simulink model "PBR_process_prod"  (R2021b)
settings: Solver=VariableStepAuto  StartTime=0.0  StopTime=300  RelTol=1e-3
values from neighbouring files (symbols this model uses):
  b = 0.0008    [PBR_estim_5_param.m]    (also in PBR_optim_orizont.m)
  D = 0    [PBR_estim_5_param.m]    (also in PBR_optim_orizont.m = linspace(0,0.1,100))
  Ea = 200    [PBR_estim_5_param.m]    (also in PBR_optim_orizont.m)
  Es = 870    [PBR_estim_5_param.m]    (also in PBR_optim_orizont.m)
  I0 = 500    [PBR_estim_5_param.m]    (also in PBR_optim_orizont.m)
  Kn = params(3)    [PBR_estim_5_param.m]    (also in PBR_optim_orizont.m = 0.13236)
  Ks = params(2)    [PBR_estim_5_param.m]    (also in PBR_optim_orizont.m = 101.2637)
  L = 0.054    [PBR_estim_5_param.m]    (also in PBR_optim_orizont.m)
  mud = params(5)    [PBR_estim_5_param.m]    (also in PBR_optim_orizont.m = 0.010177)
  mumax = params(1)    [PBR_estim_5_param.m]    (also in PBR_optim_orizont.m = 0.21692)
  N0 = 2    [PBR_estim_5_param.m]    (also in PBR_optim_orizont.m = 1.5)
  Nin = 1    [PBR_estim_5_param.m]    (also in PBR_optim_orizont.m = 2)
  X0 = 0.1    [PBR_estim_5_param.m]    (also in PBR_optim_orizont.m)
  Ynx = params(4)    [PBR_estim_5_param.m]    (also in PBR_optim_orizont.m = 0.043508)
settings Model: Creator=georg
settings SolverCC: AlgebraicLoopSolver=TrustRegion
settings DataIOCC: ReturnWorkspaceOutputs=off
settings DebuggingCC: ArithmeticOperatorsInVariantConditions=warning
settings SFSimCC: CustomCodeUndefinedFunction=UseInterfaceOnly
settings RTWCC: DLArmComputeVersion=20.02.1

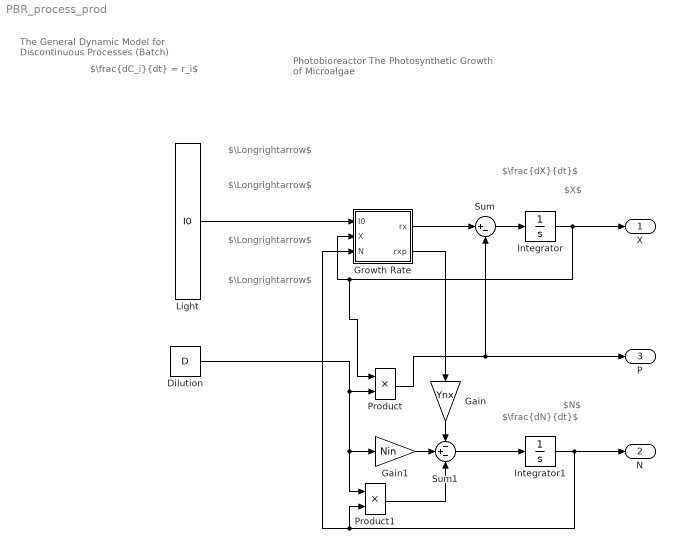
== system PBR_process_prod ==
  note: Photobioreactor
      | The Photosynthetic Growth of Microalgae
  note: $X$
  note: $\frac{dX}{dt}$
  note: $\Longrightarrow$
  note: $\Longrightarrow$
  note: $\frac{dC_i}{dt} = r_i$
  note: $\Longrightarrow$
  note: The General Dynamic Model for
      | Discontinuous Processes (Batch)
  note: $\Longrightarrow$
  note: $\frac{dN}{dt}$
  note: $N$
  Dilution : Constant  Value=D
  Gain : Gain  Gain=Ynx
  Gain1 : Gain  Gain=Nin
  Growth Rate : Subsystem
  Integrator : Integrator  InitialCondition=X0
  Integrator1 : Integrator  InitialCondition=N0
  Light : Constant  Value=I0
  Product : Product
  Product1 : Product
  Sum : Sum  Inputs=|+-
  Sum1 : Sum  Inputs=-+-
  X : Outport
  N : Outport  Port=2
  P : Outport  Port=3
  wires:
  Sum/1 -> Integrator/1
  Integrator/1 -> X/1, Growth Rate/2(X), Product/1
  Growth Rate/1(rx) -> Sum/1
  Gain1/1 -> Sum1/2
  Product1/1 -> Sum1/3
  Integrator1/1 -> N/1, Growth Rate/3(N), Product1/2
  Sum1/1 -> Integrator1/1
  Gain/1 -> Sum1/1
  Growth Rate/2(rxp) -> Gain/1
  Light/1 -> Growth Rate/1(I0)
  Dilution/1 -> Gain1/1, Product1/1, Product/2
  Product/1 -> P/1, Sum/2

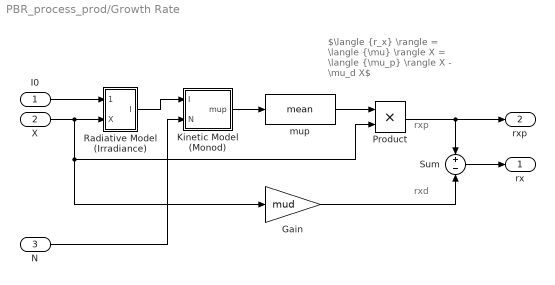
== system PBR_process_prod/Growth Rate ==
  note: $\langle {r_x} \rangle = \langle {\mu} \rangle X = \langle {\mu_p} \rangle X - \mu_d X$
  note: rxd
  note: rxp
  I0 : Inport
  X : Inport  Port=2
  N : Inport  Port=3
  Gain : Gain  Gain=mud
  Kinetic Model (Monod) : Subsystem
  Product : Product
  Radiative Model (Irradiance) : Subsystem
  Sum : Sum  Inputs=+-
  mup : MATLABFcn  MATLABFcn=mean
  rx : Outport  VectorParamsAs1DForOutWhenUnconnected=off
  rxp : Outport  Port=2  VectorParamsAs1DForOutWhenUnconnected=off
  wires:
  X/1 -> Product/2, Gain/1, Radiative Model (Irradiance)/2(X)
  Gain/1 -> Sum/2
  Sum/1 -> rx/1
  I0/1 -> Radiative Model (Irradiance)/1(I0)
  Kinetic Model (Monod)/1(mup) -> mup/1
  Radiative Model (Irradiance)/1(I) -> Kinetic Model (Monod)/1(I)
  mup/1 -> Product/1
  Product/1 -> Sum/1, rxp/1
  N/1 -> Kinetic Model (Monod)/2(N)

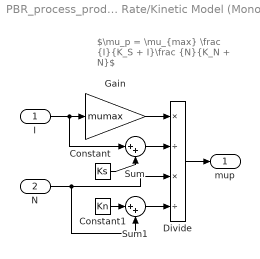
== system PBR_process_prod/Growth Rate/Kinetic Model (Monod) ==
  note: $\mu_p = \mu_{max} \frac {I}{K_S + I}\frac {N}{K_N + N}$
  I : Inport
  N : Inport  Port=2
  Constant : Constant  Value=Ks
  Constant1 : Constant  Value=Kn
  Divide : Product  Inputs=*/*/
  Gain : Gain  Gain=mumax
  Sum : Sum  Inputs=|++
  Sum1 : Sum  Inputs=|++
  mup : Outport  VectorParamsAs1DForOutWhenUnconnected=off
  wires:
  Constant/1 -> Sum/2
  Sum/1 -> Divide/2
  I/1 -> Sum/1, Gain/1
  Gain/1 -> Divide/1
  Divide/1 -> mup/1
  N/1 -> Sum1/2, Divide/3
  Sum1/1 -> Divide/4
  Constant1/1 -> Sum1/1

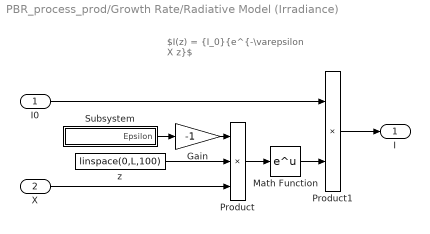
== system PBR_process_prod/Growth Rate/Radiative Model (Irradiance) ==
  note: $I(z) = {I_0}{e^{-\varepsilon X z}$
  I0 : Inport
  X : Inport  Port=2
  Gain : Gain  Gain=-1
  Math Function : Math  SignedPower=on  SaturateOnIntegerOverflow=on
  Product : Product  Inputs=3
  Product1 : Product
  Subsystem : Subsystem
  z : Constant  Value=linspace(0,L,100)
  I : Outport  VectorParamsAs1DForOutWhenUnconnected=off
  wires:
  Gain/1 -> Product/1
  Subsystem/1(Epsilon) -> Gain/1
  I0/1 -> Product1/1
  z/1 -> Product/2
  X/1 -> Product/3
  Math Function/1 -> Product1/2
  Product1/1 -> I/1
  Product/1 -> Math Function/1

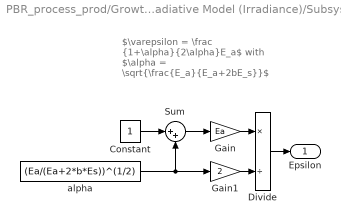
== system PBR_process_prod/Growth Rate/Radiative Model (Irradiance)/Subsystem ==
  note: $\varepsilon = \frac {1+\alpha}{2\alpha}E_a$ with $\alpha = \sqrt{\frac{E_a}{E_a+2bE_s}}$
  Constant : Constant
  Divide : Product  Inputs=*/
  Gain : Gain  Gain=Ea
  Gain1 : Gain  Gain=2
  Sum : Sum  Inputs=|++
  alpha : Constant  Value=(Ea/(Ea+2*b*Es))^(1/2)
  Epsilon : Outport  VectorParamsAs1DForOutWhenUnconnected=off
  wires:
  Gain1/1 -> Divide/2
  Constant/1 -> Sum/1
  Sum/1 -> Gain/1
  alpha/1 -> Sum/2, Gain1/1
  Gain/1 -> Divide/1
  Divide/1 -> Epsilon/1
